simulink model "MCC"  (R2017b)
settings: Solver=ode15s  StartTime=0.0  StopTime=0.2  RelTol=1e-3
values from neighbouring files (symbols this model uses):
  b = 3.5077e-6    (= 3.5077e-06)    [MCC_variables.m]    (also in TD2_config.m = 0.0085)
  Cr = 0    [MCC_variables.m]    (also in TD3.m)
  J = 3.2284e-6    (= 3.2284e-06)    [MCC_variables.m]    (also in TD2_config.m = 0.28; TD3.m = 0.2)
  Ke = K    (= 0.0274)    [MCC_variables.m]
  Kt = K    (= 0.0274)    [MCC_variables.m]
  L = 2.75e-6    (= 2.75e-06)    [MCC_variables.m]    (also in TD2_config.m = 0.0016)
  R = 4    [MCC_variables.m]    (also in TD2_config.m = 0.13; TD3.m = 0.895)
  U = 12    [MCC_variables.m]
settings Model: Creator=Table2  LastModifiedBy=Table2

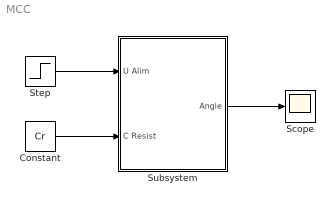
== system MCC ==
  Constant : Constant  Value=Cr
  Scope : Scope
  Step : Step  Time=0  After=U  SampleTime=0
  Subsystem : Subsystem
  wires:
  Step/1 -> Subsystem/1(U Alim)
  Constant/1 -> Subsystem/2(C Resist)
  Subsystem/1(Angle) -> Scope/1

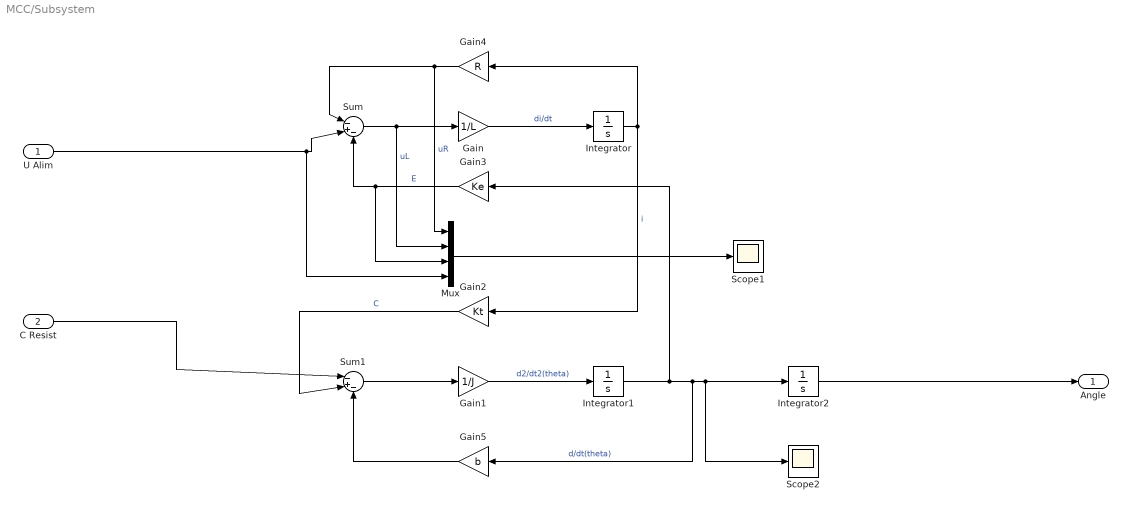
== system MCC/Subsystem ==
  U Alim : Inport
  C Resist : Inport  Port=2
  Gain : Gain  Gain=1/L
  Gain1 : Gain  Gain=1/J
  Gain2 : Gain  Gain=Kt
  Gain3 : Gain  Gain=Ke
  Gain4 : Gain  Gain=R
  Gain5 : Gain  Gain=b
  Integrator : Integrator
  Integrator1 : Integrator
  Integrator2 : Integrator
  Mux : Mux
  Scope1 : Scope
  Scope2 : Scope
  Sum : Sum  Inputs=|-+-
  Sum1 : Sum  Inputs=|-+-
  Angle : Outport
  wires:
  Integrator/1 -> Gain4/1, Gain2/1  "i"
  Gain2/1 -> Sum1/2  "C"
  Integrator1/1 -> Gain3/1, Gain5/1, Scope2/1, Integrator2/1  "d/dt(theta)"
  Gain1/1 -> Integrator1/1  "d2/dt2(theta)"
  Sum1/1 -> Gain1/1
  Gain3/1 -> Mux/3, Sum/3  "E"
  U Alim/1 -> Mux/4, Sum/2
  Gain4/1 -> Mux/1, Sum/1  "uR"
  C Resist/1 -> Sum1/1
  Gain/1 -> Integrator/1  "di/dt"
  Sum/1 -> Mux/2, Gain/1  "uL"
  Gain5/1 -> Sum1/3
  Integrator2/1 -> Angle/1
  Mux/1 -> Scope1/1
